simulink model "fig1_check_step_resp_char"  (R2016b)
settings: Solver=VariableStepAuto  StartTime=0.0  StopTime=10.0  RelTol=1e-3
values from neighbouring files (symbols this model uses):
  K = K_array(i)    [Lab2.m]    (also in lab2.m)
libraries: checkpacklib x1
settings Model: Creator=ee105-abq  LastModifiedBy=ee105-abq

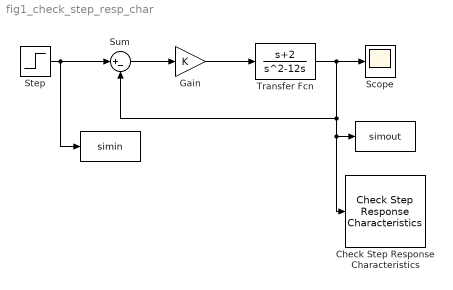
== system fig1_check_step_resp_char ==
  " " : ToWorkspace  VariableName=simout  SaveFormat=Timeseries  SampleTime=-1
  "  " : ToWorkspace  VariableName=simin  SaveFormat=Timeseries  SampleTime=-1
  Check Step Response Characteristics : checkpacklib/Check Step Response  Characteristics  InstantiateOnLoad=on  enabled=on  stopWhenAssertionFail=off  export=off  ViewDlgPos=[]  OpenViewOnLoad=off  LaunchViewOnOpen=off  TimeUnits=seconds  EnableStepResponseBound=on  InitialValue=0  FinalValue=1  StepTime=0  RiseTime=5  PercentRise=80  SettlingTime=7  PercentSettling=1  PercentOvershoot=10  PercentUndershoot=1
  Gain : Gain  Gain=K
  Scope : Scope
  Step : Step  SampleTime=0
  Sum : Sum  Inputs=|+-
  Transfer Fcn : TransferFcn  Numerator=[1 2]  Denominator=[1 -12 0]
  wires:
  Step/1 -> "  "/1, Sum/1
  Sum/1 -> Gain/1
  Gain/1 -> Transfer Fcn/1
  Transfer Fcn/1 -> Sum/2, Check Step Response Characteristics/1, " "/1, Scope/1
